simulink model "programming_simulink_bench"  (R2021b)
settings: Solver=ode1  StartTime=0.0  StopTime=120  FixedStep=0.01  RelTol=1e-3  EnableMultiTasking=on
undefined symbols (not defined in the file): a, b, c, ki, kp
libraries: arduinolib x12, arduinosensorlib x3
settings Model: ExtModeTrigDuration=2  Creator=Admin  LastModifiedBy=ASUS
settings SolverCC: AlgebraicLoopSolver=TrustRegion
settings OptimizationCC: EnhancedBackFolding=on  PassReuseOutputArgsAs=Individual arguments  ZeroExternalMemoryAtStartup=off  ZeroInternalMemoryAtStartup=off  MaxStackSize=64  OptimizeBlockOrder=speed  DifferentSizesBufferReuse=on  OptimizationCustomize=off  EfficientTunableParamExpr=on
settings DebuggingCC: ParameterTunabilityLossMsg=error  SFMachineParentedDataDiag=warning
settings HardwareCC: ProdBitPerInt=16  ProdBitPerPointer=16  ProdBitPerSizeT=16  ProdBitPerPtrDiffT=16  ProdLargestAtomicFloat=None  ProdWordSize=8  ProdHWDeviceType=Atmel->AVR
settings SFSimCC: MATLABDynamicMemAlloc=off
settings RTWCC: Description=Embedded Coder  SystemTargetFile=ert.tlc  HardwareBoard=Arduino Mega 2560  TemplateMakefile=ert_default_tmf  Toolchain=Arduino AVR  BuildConfiguration=Faster Runs
settings CodeAppCC: ForceParamTrailComments=on  IgnoreCustomStorageClasses=off  OperatorAnnotations=on  SimulinkDataObjDesc=on  SFDataObjDesc=on  InsertBlockDesc=on
settings ERTTargetCC: SupportContinuousTime=on  SupportNonInlinedSFcns=on  SupportVariableSizeSignals=on  ExtModeTransport=3  ExtModeStaticAlloc=on  ExtModeStaticAllocSize=2048  ExtModeMexFile=ext_xcp  ExtModeIntrfLevel=Level2 - Open

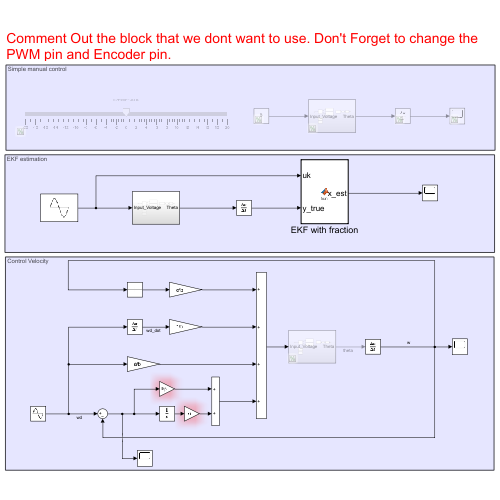
[thumbnail: Simulink's stored preview of the top-level diagram]
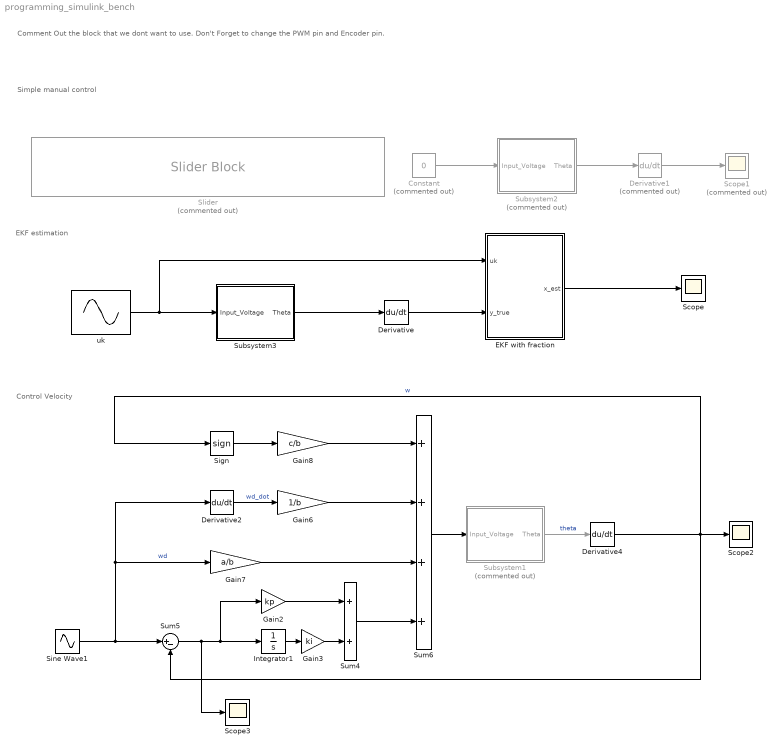
== system programming_simulink_bench ==
  note: Control Velocity
  note: Comment Out the block that we dont want to use. Don't Forget to change the PWM pin and Encoder pin.
  note: EKF estimation
  note: Simple manual control
  Constant : Constant  Commented=on  Value=0
  Derivative : Derivative
  Derivative1 : Derivative  Commented=on
  Derivative2 : Derivative
  Derivative4 : Derivative
  EKF with fraction : MATLAB Function  TreatAsAtomicUnit=on
  Gain2 : Gain  Gain=kp
  Gain3 : Gain  Gain=ki
  Gain6 : Gain  Gain=1/b
  Gain7 : Gain  Gain=a/b
  Gain8 : Gain  Gain=c/b
  Integrator1 : Integrator
  Scope : Scope
  Scope1 : Scope  Commented=on
  Scope2 : Scope
  Scope3 : Scope
  Sign : Signum
  Sine Wave1 : Sin  Amplitude=10  Frequency=2*pi*0.1  SampleTime=0
  Slider : SliderBlock  Commented=on  ScaleMin=-20  ScaleMax=20  TickInterval=2
  Subsystem1 : Subsystem  Commented=on
  Subsystem2 : Subsystem  Commented=on
  Subsystem3 : Subsystem
  Sum4 : Sum
  Sum5 : Sum  Inputs=|+-
  Sum6 : Sum  Inputs=++++
  uk : Sin  Amplitude=20  Frequency=2*pi*0.4  SampleTime=0
  wires:
  EKF with fraction/1(x_est) -> Scope/1
  Derivative/1 -> EKF with fraction/2(y_true)
  Subsystem3/1(Theta) -> Derivative/1
  uk/1 -> EKF with fraction/1(uk), Subsystem3/1(Input_Voltage)
  Constant/1 -> Subsystem2/1(Input_Voltage)
  Subsystem2/1(Theta) -> Derivative1/1
  Derivative1/1 -> Scope1/1
  Sign/1 -> Gain8/1
  Subsystem1/1(Theta) -> Derivative4/1  "theta"
  Gain6/1 -> Sum6/2
  Sum6/1 -> Subsystem1/1(Input_Voltage)
  Integrator1/1 -> Gain3/1
  Sum4/1 -> Sum6/4
  Gain8/1 -> Sum6/1
  Gain2/1 -> Sum4/1
  Sum5/1 -> Gain2/1, Integrator1/1, Scope3/1
  Derivative4/1 -> Sign/1, Sum5/2, Scope2/1  "w"
  Gain7/1 -> Sum6/3
  Sine Wave1/1 -> Sum5/1, Gain7/1, Derivative2/1  "wd"
  Gain3/1 -> Sum4/2
  Derivative2/1 -> Gain6/1  "wd_dot"

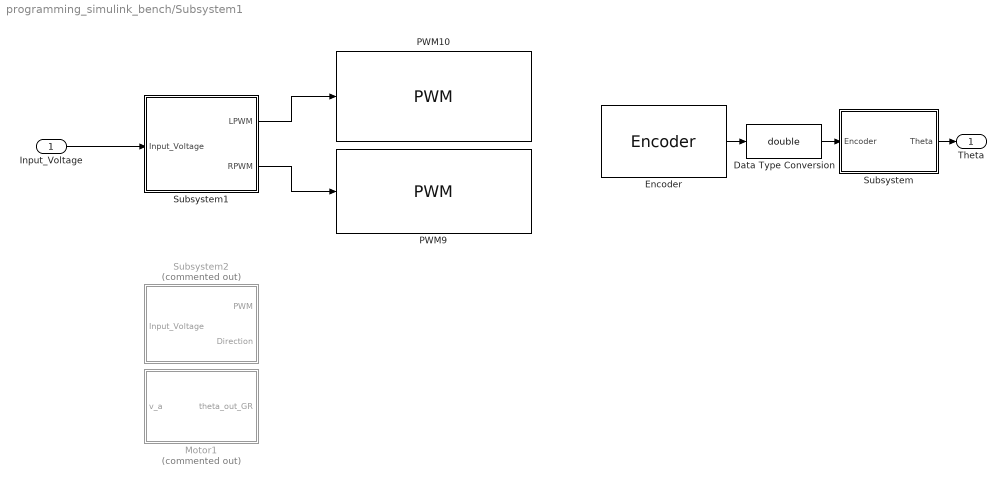
== system programming_simulink_bench/Subsystem1 ==
  Input_Voltage : Inport
  Data Type Conversion : DataTypeConversion  OutDataTypeStr=double
  Encoder : arduinosensorlib/Encoder  InputA=2  InputB=3  Mode=No reset  SampleTime=-1
      settings: SourceProductBaseCode=ARDUINO
  Motor1 : Subsystem  Commented=on
  PWM10 : arduinolib/PWM  pinNumber=8  frequencyType=Default  desiredFrequency=490.2  achievableFrequency=490.2
  PWM9 : arduinolib/PWM  pinNumber=9  frequencyType=Default  desiredFrequency=490.2  achievableFrequency=490.2
  Subsystem : Subsystem  mask(Encoder Pulse to Radian Conversion){PPR=11, Mode=1, GR=515}
      mask prompts: PPR "Base Pulse per Revolution :"; Mode "Encoder Count Mode :"; GR "Gear Box Ratio :"
      mask help: This block is used for converting motor encoder pulse to shaft position theta.
      mask TypeOptions Mode: 1 | 2 | 4
  Subsystem1 : Subsystem  mask(Motor PWM Calculation for Left, Right PWM Type){max_pwm_pulse=254, voltage_max=23.5}
      mask prompts: max_pwm_pulse "Max PWM Pulse Number :"; voltage_max "Max Voltage :"
      mask help:
      | This block is used the calculate the PWM from the input voltage for motor driver with Left and Right PWM Type (IBT-2).
      |
      | - Max PWM Pulse Number used for selecting the maximum pulse for PWM. Some driver has 255 as the maximum PWM and some has 254 as the maximum.
      |
      | - Max Voltage used for input the maximum voltage for the battery and the motor. Typically, the DC Motor and battery use 24v.
      mask TypeOptions max_pwm_pulse: 254 | 255
  Subsystem2 : Subsystem  Commented=on  mask(Motor PWM Calculation for PWM, Direction Type){max_pwm_pulse=254, voltage_max=0}
      mask help:
      | This block is used the calculate the PWM from the input voltage for motor driver with PWM and Direction Type.
      |
      | - Max PWM Pulse Number used for selecting the maximum pulse for PWM. Some driver has 255 as the maximum PWM and some has 254 as the maximum.
      |
      | - Max Voltage used for input the maximum voltage for the battery and the motor. Typically, the DC Motor and battery use 24v.
      mask TypeOptions max_pwm_pulse: 254 | 255
  Theta : Outport
  wires:
  Subsystem/1(Theta) -> Theta/1
  Subsystem1/2(RPWM) -> PWM9/1
  Input_Voltage/1 -> Subsystem1/1(Input_Voltage)
  Subsystem1/1(LPWM) -> PWM10/1
  Encoder/1 -> Data Type Conversion/1
  Data Type Conversion/1 -> Subsystem/1(Encoder)

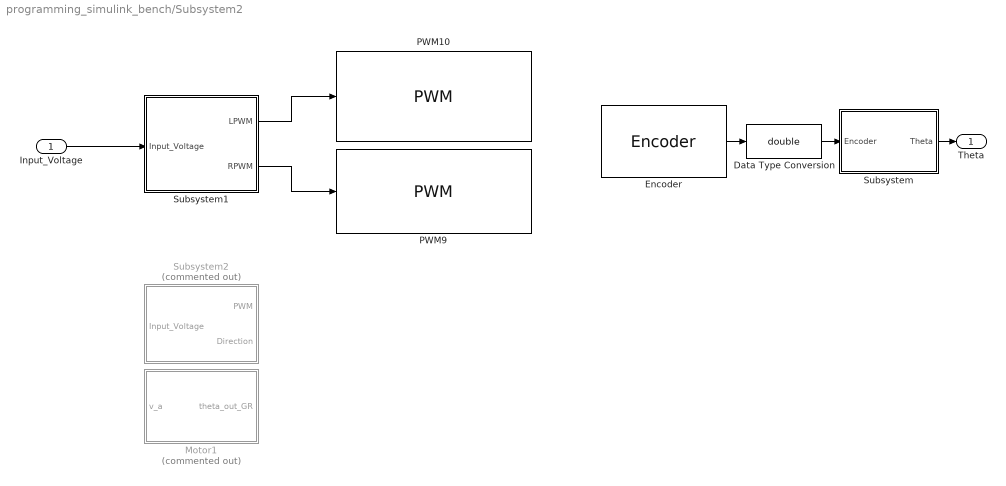
== system programming_simulink_bench/Subsystem2 ==
  Input_Voltage : Inport
  Data Type Conversion : DataTypeConversion  OutDataTypeStr=double
  Encoder : arduinosensorlib/Encoder  InputA=2  InputB=3  Mode=No reset  SampleTime=-1
      settings: SourceProductBaseCode=ARDUINO
  Motor1 : Subsystem  Commented=on
  PWM10 : arduinolib/PWM  pinNumber=8  frequencyType=Default  desiredFrequency=490.2  achievableFrequency=490.2
  PWM9 : arduinolib/PWM  pinNumber=9  frequencyType=Default  desiredFrequency=490.2  achievableFrequency=490.2
  Subsystem : Subsystem  mask(Encoder Pulse to Radian Conversion){PPR=11, Mode=1, GR=515}
      mask prompts: PPR "Base Pulse per Revolution :"; Mode "Encoder Count Mode :"; GR "Gear Box Ratio :"
      mask help: This block is used for converting motor encoder pulse to shaft position theta.
      mask TypeOptions Mode: 1 | 2 | 4
  Subsystem1 : Subsystem  mask(Motor PWM Calculation for Left, Right PWM Type){max_pwm_pulse=254, voltage_max=23.5}
      mask prompts: max_pwm_pulse "Max PWM Pulse Number :"; voltage_max "Max Voltage :"
      mask help:
      | This block is used the calculate the PWM from the input voltage for motor driver with Left and Right PWM Type (IBT-2).
      |
      | - Max PWM Pulse Number used for selecting the maximum pulse for PWM. Some driver has 255 as the maximum PWM and some has 254 as the maximum.
      |
      | - Max Voltage used for input the maximum voltage for the battery and the motor. Typically, the DC Motor and battery use 24v.
      mask TypeOptions max_pwm_pulse: 254 | 255
  Subsystem2 : Subsystem  Commented=on  mask(Motor PWM Calculation for PWM, Direction Type){max_pwm_pulse=254, voltage_max=0}
      mask help:
      | This block is used the calculate the PWM from the input voltage for motor driver with PWM and Direction Type.
      |
      | - Max PWM Pulse Number used for selecting the maximum pulse for PWM. Some driver has 255 as the maximum PWM and some has 254 as the maximum.
      |
      | - Max Voltage used for input the maximum voltage for the battery and the motor. Typically, the DC Motor and battery use 24v.
      mask TypeOptions max_pwm_pulse: 254 | 255
  Theta : Outport
  wires:
  Data Type Conversion/1 -> Subsystem/1(Encoder)
  Encoder/1 -> Data Type Conversion/1
  Subsystem1/1(LPWM) -> PWM10/1
  Input_Voltage/1 -> Subsystem1/1(Input_Voltage)
  Subsystem1/2(RPWM) -> PWM9/1
  Subsystem/1(Theta) -> Theta/1

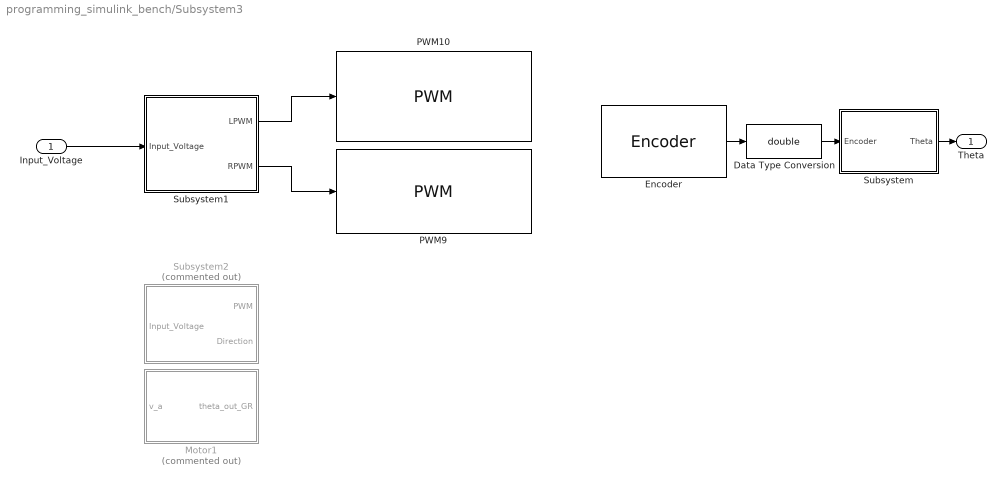
== system programming_simulink_bench/Subsystem3 ==
  Input_Voltage : Inport
  Data Type Conversion : DataTypeConversion  OutDataTypeStr=double
  Encoder : arduinosensorlib/Encoder  InputA=2  InputB=3  Mode=No reset  SampleTime=-1
      settings: SourceProductBaseCode=ARDUINO
  Motor1 : Subsystem  Commented=on
  PWM10 : arduinolib/PWM  pinNumber=8  frequencyType=Default  desiredFrequency=490.2  achievableFrequency=490.2
  PWM9 : arduinolib/PWM  pinNumber=9  frequencyType=Default  desiredFrequency=490.2  achievableFrequency=490.2
  Subsystem : Subsystem  mask(Encoder Pulse to Radian Conversion){PPR=11, Mode=1, GR=515}
      mask prompts: PPR "Base Pulse per Revolution :"; Mode "Encoder Count Mode :"; GR "Gear Box Ratio :"
      mask help: This block is used for converting motor encoder pulse to shaft position theta.
      mask TypeOptions Mode: 1 | 2 | 4
  Subsystem1 : Subsystem  mask(Motor PWM Calculation for Left, Right PWM Type){max_pwm_pulse=254, voltage_max=23.5}
      mask prompts: max_pwm_pulse "Max PWM Pulse Number :"; voltage_max "Max Voltage :"
      mask help:
      | This block is used the calculate the PWM from the input voltage for motor driver with Left and Right PWM Type (IBT-2).
      |
      | - Max PWM Pulse Number used for selecting the maximum pulse for PWM. Some driver has 255 as the maximum PWM and some has 254 as the maximum.
      |
      | - Max Voltage used for input the maximum voltage for the battery and the motor. Typically, the DC Motor and battery use 24v.
      mask TypeOptions max_pwm_pulse: 254 | 255
  Subsystem2 : Subsystem  Commented=on  mask(Motor PWM Calculation for PWM, Direction Type){max_pwm_pulse=254, voltage_max=0}
      mask help:
      | This block is used the calculate the PWM from the input voltage for motor driver with PWM and Direction Type.
      |
      | - Max PWM Pulse Number used for selecting the maximum pulse for PWM. Some driver has 255 as the maximum PWM and some has 254 as the maximum.
      |
      | - Max Voltage used for input the maximum voltage for the battery and the motor. Typically, the DC Motor and battery use 24v.
      mask TypeOptions max_pwm_pulse: 254 | 255
  Theta : Outport
  wires:
  Data Type Conversion/1 -> Subsystem/1(Encoder)
  Encoder/1 -> Data Type Conversion/1
  Subsystem1/1(LPWM) -> PWM10/1
  Input_Voltage/1 -> Subsystem1/1(Input_Voltage)
  Subsystem1/2(RPWM) -> PWM9/1
  Subsystem/1(Theta) -> Theta/1

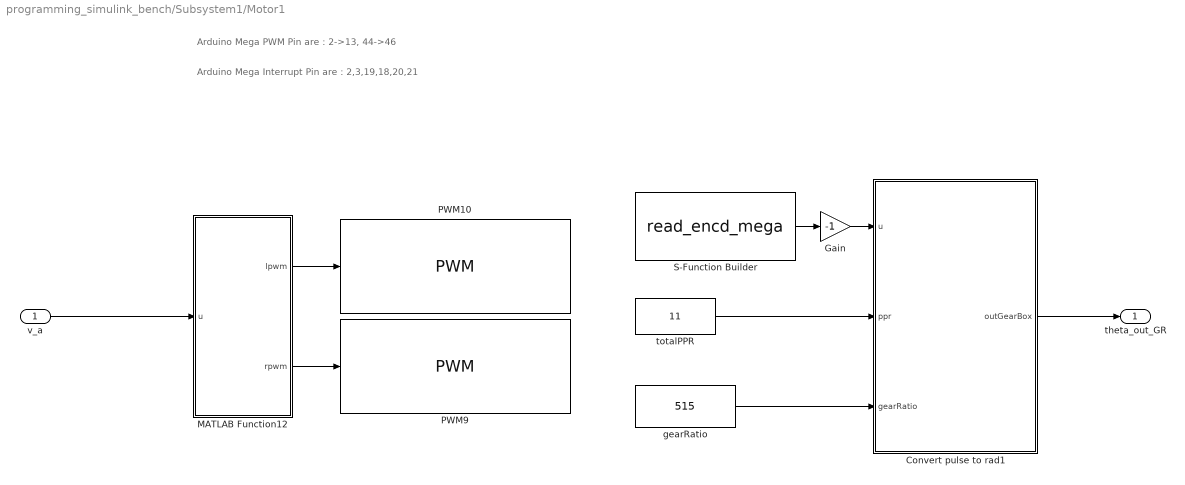
== system programming_simulink_bench/Subsystem1/Motor1 ==
  note: Arduino Mega PWM Pin are : 2->13, 44->46
  note: Arduino Mega Interrupt Pin are : 2,3,19,18,20,21
  v_a : Inport
  Convert pulse to rad1 : MATLAB Function  TreatAsAtomicUnit=on
  Gain : Gain  Gain=-1
  MATLAB Function12 : MATLAB Function  TreatAsAtomicUnit=on
  PWM10 : arduinolib/PWM  pinNumber=8  frequencyType=Default  desiredFrequency=490.2  achievableFrequency=490.2
  PWM9 : arduinolib/PWM  pinNumber=9  frequencyType=Default  desiredFrequency=490.2  achievableFrequency=490.2
  S-Function Builder : S-Function  FunctionName=read_encd_mega  SFunctionModules=read_encd_mega_wrapper  SFunctionDeploymentMode=off  EnableBusSupport=off  mask(S-Function Builder){}
      mask help: Simulink:masks:SFunctionBuilder_MD
      mask init:
      | val = [[.9  0.75 0.75 1 1 .9 .9 1]',[1 1 0.75 0.75 .9 .9 1 .9]'];try , sys = get_param(gcb,'SfunBuilderFcnName');if isempty(sys), sys = get_param(gcb,'FunctionName'); end,catch, sys = get_param(gcb,'FunctionName'); end
      settings: CopyFcn=set_param(gcbh,'LinkStatus','none')  OpenFcn=sfunctionwizard(gcbh)
      mask Display: plot(val(:,1),val(:,2)),disp(sys),port_label('output',1,'count')
  gearRatio : Constant  Value=515
  totalPPR : Constant  Value=11
  theta_out_GR : Outport
  wires:
  Gain/1 -> Convert pulse to rad1/1(u)
  S-Function Builder/1 -> Gain/1
  Convert pulse to rad1/1(outGearBox) -> theta_out_GR/1
  v_a/1 -> MATLAB Function12/1(u)
  gearRatio/1 -> Convert pulse to rad1/3(gearRatio)
  MATLAB Function12/2(rpwm) -> PWM9/1
  totalPPR/1 -> Convert pulse to rad1/2(ppr)
  MATLAB Function12/1(lpwm) -> PWM10/1

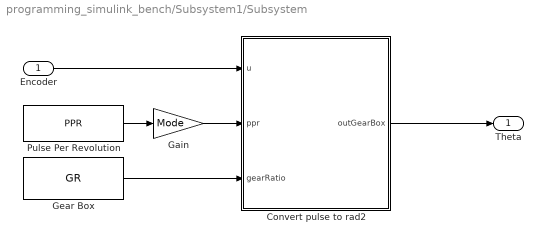
== system programming_simulink_bench/Subsystem1/Subsystem ==
  Encoder : Inport
  Convert pulse to rad2 : MATLAB Function  TreatAsAtomicUnit=on
  Gain : Gain  Gain=Mode
  Gear Box : Constant  Value=GR
  Pulse Per Revolution : Constant  Value=PPR
  Theta : Outport
  wires:
  Gain/1 -> Convert pulse to rad2/2(ppr)
  Encoder/1 -> Convert pulse to rad2/1(u)
  Gear Box/1 -> Convert pulse to rad2/3(gearRatio)
  Pulse Per Revolution/1 -> Gain/1
  Convert pulse to rad2/1(outGearBox) -> Theta/1

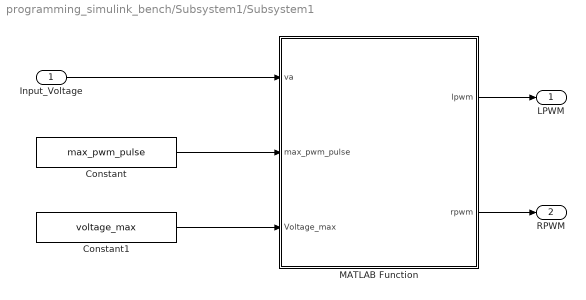
== system programming_simulink_bench/Subsystem1/Subsystem1 ==
  Input_Voltage : Inport
  Constant : Constant  Value=max_pwm_pulse
  Constant1 : Constant  Value=voltage_max
  MATLAB Function : MATLAB Function  TreatAsAtomicUnit=on
  LPWM : Outport
  RPWM : Outport  Port=2
  wires:
  Input_Voltage/1 -> MATLAB Function/1(va)
  MATLAB Function/1(lpwm) -> LPWM/1
  Constant1/1 -> MATLAB Function/3(Voltage_max)
  Constant/1 -> MATLAB Function/2(max_pwm_pulse)
  MATLAB Function/2(rpwm) -> RPWM/1

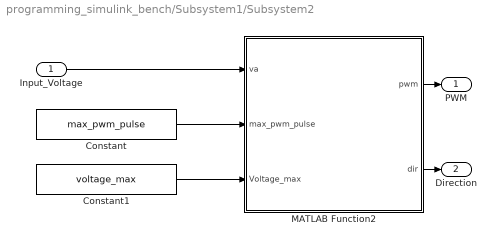
== system programming_simulink_bench/Subsystem1/Subsystem2 ==
  Input_Voltage : Inport
  Constant : Constant  Value=max_pwm_pulse
  Constant1 : Constant  Value=voltage_max
  MATLAB Function2 : MATLAB Function  TreatAsAtomicUnit=on
  PWM : Outport
  Direction : Outport  Port=2
  wires:
  MATLAB Function2/1(pwm) -> PWM/1
  Input_Voltage/1 -> MATLAB Function2/1(va)
  MATLAB Function2/2(dir) -> Direction/1
  Constant1/1 -> MATLAB Function2/3(Voltage_max)
  Constant/1 -> MATLAB Function2/2(max_pwm_pulse)

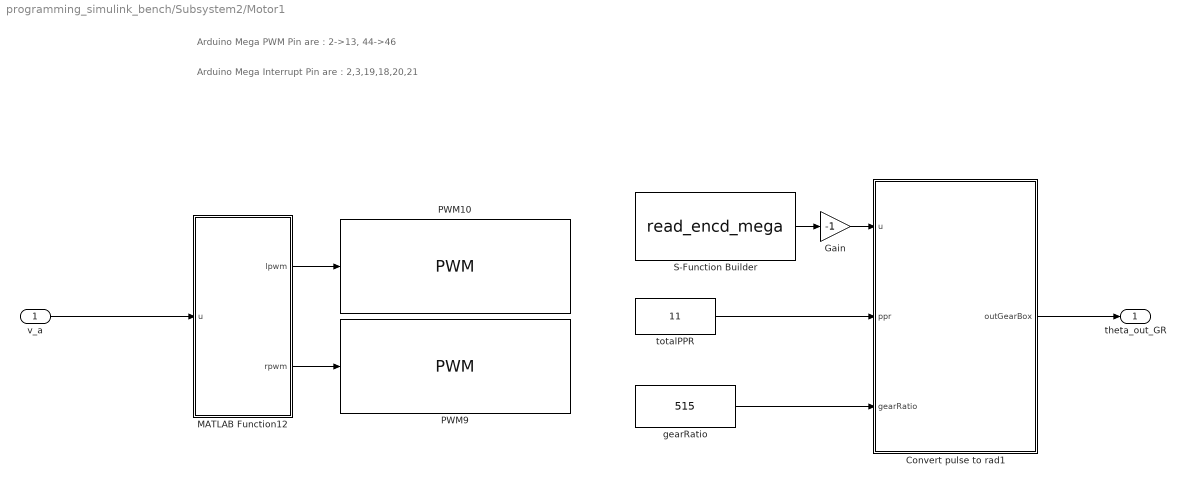
== system programming_simulink_bench/Subsystem2/Motor1 ==
  note: Arduino Mega Interrupt Pin are : 2,3,19,18,20,21
  note: Arduino Mega PWM Pin are : 2->13, 44->46
  v_a : Inport
  Convert pulse to rad1 : MATLAB Function  TreatAsAtomicUnit=on
  Gain : Gain  Gain=-1
  MATLAB Function12 : MATLAB Function  TreatAsAtomicUnit=on
  PWM10 : arduinolib/PWM  pinNumber=8  frequencyType=Default  desiredFrequency=490.2  achievableFrequency=490.2
  PWM9 : arduinolib/PWM  pinNumber=9  frequencyType=Default  desiredFrequency=490.2  achievableFrequency=490.2
  S-Function Builder : S-Function  FunctionName=read_encd_mega  SFunctionModules=read_encd_mega_wrapper  SFunctionDeploymentMode=off  EnableBusSupport=off  mask(S-Function Builder){}
      mask help: Simulink:masks:SFunctionBuilder_MD
      mask init: same as programming_simulink_bench/Subsystem1/Motor1/S-Function Builder
      settings: CopyFcn=set_param(gcbh,'LinkStatus','none')  OpenFcn=sfunctionwizard(gcbh)
      mask Display: plot(val(:,1),val(:,2)),disp(sys),port_label('output',1,'count')
  gearRatio : Constant  Value=515
  totalPPR : Constant  Value=11
  theta_out_GR : Outport
  wires:
  MATLAB Function12/1(lpwm) -> PWM10/1
  totalPPR/1 -> Convert pulse to rad1/2(ppr)
  MATLAB Function12/2(rpwm) -> PWM9/1
  gearRatio/1 -> Convert pulse to rad1/3(gearRatio)
  v_a/1 -> MATLAB Function12/1(u)
  Convert pulse to rad1/1(outGearBox) -> theta_out_GR/1
  S-Function Builder/1 -> Gain/1
  Gain/1 -> Convert pulse to rad1/1(u)

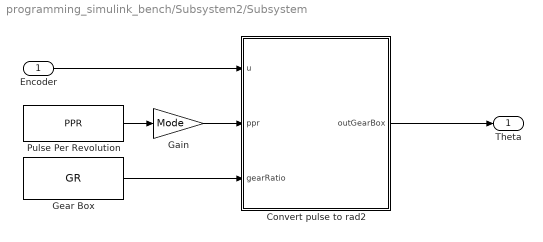
== system programming_simulink_bench/Subsystem2/Subsystem ==
  Encoder : Inport
  Convert pulse to rad2 : MATLAB Function  TreatAsAtomicUnit=on
  Gain : Gain  Gain=Mode
  Gear Box : Constant  Value=GR
  Pulse Per Revolution : Constant  Value=PPR
  Theta : Outport
  wires:
  Convert pulse to rad2/1(outGearBox) -> Theta/1
  Pulse Per Revolution/1 -> Gain/1
  Gear Box/1 -> Convert pulse to rad2/3(gearRatio)
  Encoder/1 -> Convert pulse to rad2/1(u)
  Gain/1 -> Convert pulse to rad2/2(ppr)

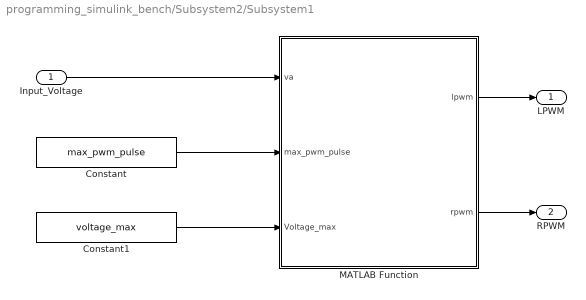
== system programming_simulink_bench/Subsystem2/Subsystem1 ==
  Input_Voltage : Inport
  Constant : Constant  Value=max_pwm_pulse
  Constant1 : Constant  Value=voltage_max
  MATLAB Function : MATLAB Function  TreatAsAtomicUnit=on
  LPWM : Outport
  RPWM : Outport  Port=2
  wires:
  MATLAB Function/2(rpwm) -> RPWM/1
  Constant/1 -> MATLAB Function/2(max_pwm_pulse)
  Constant1/1 -> MATLAB Function/3(Voltage_max)
  MATLAB Function/1(lpwm) -> LPWM/1
  Input_Voltage/1 -> MATLAB Function/1(va)

== system programming_simulink_bench/Subsystem2/Subsystem2 ==
  Input_Voltage : Inport
  Constant : Constant  Value=max_pwm_pulse
  Constant1 : Constant  Value=voltage_max
  MATLAB Function2 : MATLAB Function  TreatAsAtomicUnit=on
  PWM : Outport
  Direction : Outport  Port=2
  wires:
  Constant/1 -> MATLAB Function2/2(max_pwm_pulse)
  Constant1/1 -> MATLAB Function2/3(Voltage_max)
  MATLAB Function2/2(dir) -> Direction/1
  Input_Voltage/1 -> MATLAB Function2/1(va)
  MATLAB Function2/1(pwm) -> PWM/1

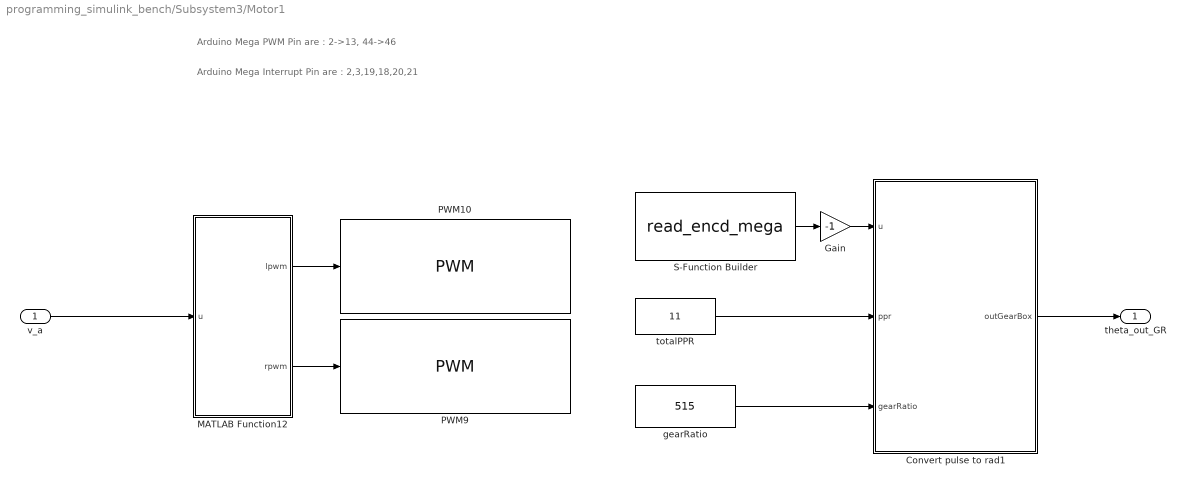
== system programming_simulink_bench/Subsystem3/Motor1 ==
  note: Arduino Mega Interrupt Pin are : 2,3,19,18,20,21
  note: Arduino Mega PWM Pin are : 2->13, 44->46
  v_a : Inport
  Convert pulse to rad1 : MATLAB Function  TreatAsAtomicUnit=on
  Gain : Gain  Gain=-1
  MATLAB Function12 : MATLAB Function  TreatAsAtomicUnit=on
  PWM10 : arduinolib/PWM  pinNumber=8  frequencyType=Default  desiredFrequency=490.2  achievableFrequency=490.2
  PWM9 : arduinolib/PWM  pinNumber=9  frequencyType=Default  desiredFrequency=490.2  achievableFrequency=490.2
  S-Function Builder : S-Function  FunctionName=read_encd_mega  SFunctionModules=read_encd_mega_wrapper  SFunctionDeploymentMode=off  EnableBusSupport=off  mask(S-Function Builder){}
      mask help: Simulink:masks:SFunctionBuilder_MD
      mask init: same as programming_simulink_bench/Subsystem1/Motor1/S-Function Builder
      settings: CopyFcn=set_param(gcbh,'LinkStatus','none')  OpenFcn=sfunctionwizard(gcbh)
      mask Display: plot(val(:,1),val(:,2)),disp(sys),port_label('output',1,'count')
  gearRatio : Constant  Value=515
  totalPPR : Constant  Value=11
  theta_out_GR : Outport
  wires:
  MATLAB Function12/1(lpwm) -> PWM10/1
  totalPPR/1 -> Convert pulse to rad1/2(ppr)
  MATLAB Function12/2(rpwm) -> PWM9/1
  gearRatio/1 -> Convert pulse to rad1/3(gearRatio)
  v_a/1 -> MATLAB Function12/1(u)
  Convert pulse to rad1/1(outGearBox) -> theta_out_GR/1
  S-Function Builder/1 -> Gain/1
  Gain/1 -> Convert pulse to rad1/1(u)

== system programming_simulink_bench/Subsystem3/Subsystem ==
  Encoder : Inport
  Convert pulse to rad2 : MATLAB Function  TreatAsAtomicUnit=on
  Gain : Gain  Gain=Mode
  Gear Box : Constant  Value=GR
  Pulse Per Revolution : Constant  Value=PPR
  Theta : Outport
  wires:
  Convert pulse to rad2/1(outGearBox) -> Theta/1
  Pulse Per Revolution/1 -> Gain/1
  Gear Box/1 -> Convert pulse to rad2/3(gearRatio)
  Encoder/1 -> Convert pulse to rad2/1(u)
  Gain/1 -> Convert pulse to rad2/2(ppr)

== system programming_simulink_bench/Subsystem3/Subsystem1 ==
  Input_Voltage : Inport
  Constant : Constant  Value=max_pwm_pulse
  Constant1 : Constant  Value=voltage_max
  MATLAB Function : MATLAB Function  TreatAsAtomicUnit=on
  LPWM : Outport
  RPWM : Outport  Port=2
  wires:
  MATLAB Function/2(rpwm) -> RPWM/1
  Constant/1 -> MATLAB Function/2(max_pwm_pulse)
  Constant1/1 -> MATLAB Function/3(Voltage_max)
  MATLAB Function/1(lpwm) -> LPWM/1
  Input_Voltage/1 -> MATLAB Function/1(va)

== system programming_simulink_bench/Subsystem3/Subsystem2 ==
  Input_Voltage : Inport
  Constant : Constant  Value=max_pwm_pulse
  Constant1 : Constant  Value=voltage_max
  MATLAB Function2 : MATLAB Function  TreatAsAtomicUnit=on
  PWM : Outport
  Direction : Outport  Port=2
  wires:
  Constant/1 -> MATLAB Function2/2(max_pwm_pulse)
  Constant1/1 -> MATLAB Function2/3(Voltage_max)
  MATLAB Function2/2(dir) -> Direction/1
  Input_Voltage/1 -> MATLAB Function2/1(va)
  MATLAB Function2/1(pwm) -> PWM/1

== matlab function programming_simulink_bench/Subsystem1/Subsystem2/MATLAB Function2 ==
  data: va input; pwm output; dir output; max_pwm_pulse input; Voltage_max input
function [pwm,dir] = fcn(va,max_pwm_pulse,Voltage_max)

pwm_cal = va*max_pwm_pulse/Voltage_max;
if pwm_cal > 0
    pwm = pwm_cal;
    dir = 0;
elseif pwm_cal < 0
    pwm = abs(pwm_cal);
    dir = 1;
else
    pwm = 0;
    dir = 0;
end

== matlab function programming_simulink_bench/Subsystem2/Motor1/Convert pulse to rad1 ==
  settings: updateMethod=DISCRETE
  data: u input; ppr input; gearRatio input; outGearBox output
function outGearBox = fcn(u,ppr,gearRatio)

persistent counter_num over_flag
if(isempty(counter_num)), counter_num = 0;end
if(isempty(over_flag)), over_flag = 0;end
pulse2radian = 2*pi/ppr; % 1 pulse = ?? radian

if(double(u) - counter_num > 40000), over_flag = over_flag-1;
elseif(double(u) - counter_num < -40000), over_flag = over_flag+1;
end

inGearBox = (double(u)+over_flag*(2^32 -1))*pulse2radian; 
outGearBox = inGearBox/gearRatio;
counter_num = double(u) ;

== matlab function programming_simulink_bench/EKF with fraction ==
  settings: updateMethod=DISCRETE
  data: uk input; y_true input; x_est output
function x_est = fcn(uk,y_true)
Ts=0.01;
persistent x_est_p P Qd_est R_est Qc_est;
if isempty(x_est_p)
          
          x_est_p=[2;13;25;1];
          P=2*eye(4);
         Qc_est=1e-5*diag([10,25,25,1]);
          Qd_est=Qc_est*Ts;
          R_est=0.02;
end
c=[1 0 0 0];D=0;Ck=c;Dk=D;
%Comput Kalman Gain and update predicted value
Wk=P*Ck'/(Ck*P*Ck'+R_est);
y_est=Ck*x_est_p+Dk*uk;
x=x_est_p+Wk.*(y_true-y_est);
%Compute prediction at next time step
x_est=x+Ts*[-x(2)*x(1)+uk*x(3)-x(4)*sign(x(1));0;0;0];
%Update error covariance matrices
P=P-Wk*Ck*P;
%Define Ak
Ak=eye(4)+Ts*[-x(2) -x(1) uk -sign(x(1));0 0 0 0;0 0 0 0;0 0 0 0];
P=Ak*P*Ak'+Qd_est;
x_est_p=x_est;

== matlab function programming_simulink_bench/Subsystem2/Motor1/MATLAB Function12 ==
  data: u input; lpwm output; rpwm output
function [lpwm,rpwm] = fcn(u)

Vmax = 23.5;
pwm = u*254/Vmax;
if pwm > 0
    lpwm = pwm;
    rpwm = 0;
elseif pwm < 0
    lpwm = 0;
    rpwm = abs(pwm);
else
    lpwm = 0;
    rpwm = 0;
end

== matlab function programming_simulink_bench/Subsystem2/Subsystem/Convert pulse to rad2 ==
  settings: updateMethod=DISCRETE
  data: u input; ppr input; gearRatio input; outGearBox output
function outGearBox = fcn(u,ppr,gearRatio)

persistent counter_num over_flag
if(isempty(counter_num)), counter_num = 0;end
if(isempty(over_flag)), over_flag = 0;end
pulse2radian = 2*pi/ppr; % 1 pulse = ?? radian

if(double(u) - counter_num > 40000), over_flag = over_flag-1;
elseif(double(u) - counter_num < -40000), over_flag = over_flag+1;
end

inGearBox = (double(u)+over_flag*(2^32 -1))*pulse2radian; 
outGearBox = inGearBox/gearRatio;
counter_num = double(u) ;

== matlab function programming_simulink_bench/Subsystem2/Subsystem1/MATLAB Function ==
  data: va input; lpwm output; max_pwm_pulse input; Voltage_max input; rpwm output
function [lpwm,rpwm] = fcn(va,max_pwm_pulse,Voltage_max)

pwm = va*max_pwm_pulse/Voltage_max;
if pwm > 0
    lpwm = pwm;
    rpwm = 0;
elseif pwm < 0
    lpwm = 0;
    rpwm = abs(pwm);
else
    lpwm = 0;
    rpwm = 0;
end

== matlab function programming_simulink_bench/Subsystem2/Subsystem2/MATLAB Function2 ==
  data: va input; pwm output; dir output; max_pwm_pulse input; Voltage_max input
function [pwm,dir] = fcn(va,max_pwm_pulse,Voltage_max)

pwm_cal = va*max_pwm_pulse/Voltage_max;
if pwm_cal > 0
    pwm = pwm_cal;
    dir = 0;
elseif pwm_cal < 0
    pwm = abs(pwm_cal);
    dir = 1;
else
    pwm = 0;
    dir = 0;
end

== matlab function programming_simulink_bench/Subsystem1/Motor1/Convert pulse to rad1 ==
  settings: updateMethod=DISCRETE
  data: u input; ppr input; gearRatio input; outGearBox output
function outGearBox = fcn(u,ppr,gearRatio)

persistent counter_num over_flag
if(isempty(counter_num)), counter_num = 0;end
if(isempty(over_flag)), over_flag = 0;end
pulse2radian = 2*pi/ppr; % 1 pulse = ?? radian

if(double(u) - counter_num > 40000), over_flag = over_flag-1;
elseif(double(u) - counter_num < -40000), over_flag = over_flag+1;
end

inGearBox = (double(u)+over_flag*(2^32 -1))*pulse2radian; 
outGearBox = inGearBox/gearRatio;
counter_num = double(u) ;

== matlab function programming_simulink_bench/Subsystem3/Motor1/Convert pulse to rad1 ==
  settings: updateMethod=DISCRETE
  data: u input; ppr input; gearRatio input; outGearBox output
function outGearBox = fcn(u,ppr,gearRatio)

persistent counter_num over_flag
if(isempty(counter_num)), counter_num = 0;end
if(isempty(over_flag)), over_flag = 0;end
pulse2radian = 2*pi/ppr; % 1 pulse = ?? radian

if(double(u) - counter_num > 40000), over_flag = over_flag-1;
elseif(double(u) - counter_num < -40000), over_flag = over_flag+1;
end

inGearBox = (double(u)+over_flag*(2^32 -1))*pulse2radian; 
outGearBox = inGearBox/gearRatio;
counter_num = double(u) ;

== matlab function programming_simulink_bench/Subsystem1/Motor1/MATLAB Function12 ==
  data: u input; lpwm output; rpwm output
function [lpwm,rpwm] = fcn(u)

Vmax = 23.5;
pwm = u*254/Vmax;
if pwm > 0
    lpwm = pwm;
    rpwm = 0;
elseif pwm < 0
    lpwm = 0;
    rpwm = abs(pwm);
else
    lpwm = 0;
    rpwm = 0;
end

== matlab function programming_simulink_bench/Subsystem3/Motor1/MATLAB Function12 ==
  data: u input; lpwm output; rpwm output
function [lpwm,rpwm] = fcn(u)

Vmax = 23.5;
pwm = u*254/Vmax;
if pwm > 0
    lpwm = pwm;
    rpwm = 0;
elseif pwm < 0
    lpwm = 0;
    rpwm = abs(pwm);
else
    lpwm = 0;
    rpwm = 0;
end

== matlab function programming_simulink_bench/Subsystem3/Subsystem/Convert pulse to rad2 ==
  settings: updateMethod=DISCRETE
  data: u input; ppr input; gearRatio input; outGearBox output
function outGearBox = fcn(u,ppr,gearRatio)

persistent counter_num over_flag
if(isempty(counter_num)), counter_num = 0;end
if(isempty(over_flag)), over_flag = 0;end
pulse2radian = 2*pi/ppr; % 1 pulse = ?? radian

if(double(u) - counter_num > 40000), over_flag = over_flag-1;
elseif(double(u) - counter_num < -40000), over_flag = over_flag+1;
end

inGearBox = (double(u)+over_flag*(2^32 -1))*pulse2radian; 
outGearBox = inGearBox/gearRatio;
counter_num = double(u) ;

== matlab function programming_simulink_bench/Subsystem3/Subsystem1/MATLAB Function ==
  data: va input; lpwm output; max_pwm_pulse input; Voltage_max input; rpwm output
function [lpwm,rpwm] = fcn(va,max_pwm_pulse,Voltage_max)

pwm = va*max_pwm_pulse/Voltage_max;
if pwm > 0
    lpwm = pwm;
    rpwm = 0;
elseif pwm < 0
    lpwm = 0;
    rpwm = abs(pwm);
else
    lpwm = 0;
    rpwm = 0;
end

== matlab function programming_simulink_bench/Subsystem3/Subsystem2/MATLAB Function2 ==
  data: va input; pwm output; dir output; max_pwm_pulse input; Voltage_max input
function [pwm,dir] = fcn(va,max_pwm_pulse,Voltage_max)

pwm_cal = va*max_pwm_pulse/Voltage_max;
if pwm_cal > 0
    pwm = pwm_cal;
    dir = 0;
elseif pwm_cal < 0
    pwm = abs(pwm_cal);
    dir = 1;
else
    pwm = 0;
    dir = 0;
end

== matlab function programming_simulink_bench/Subsystem1/Subsystem/Convert pulse to rad2 ==
  settings: updateMethod=DISCRETE
  data: u input; ppr input; gearRatio input; outGearBox output
function outGearBox = fcn(u,ppr,gearRatio)

persistent counter_num over_flag
if(isempty(counter_num)), counter_num = 0;end
if(isempty(over_flag)), over_flag = 0;end
pulse2radian = 2*pi/ppr; % 1 pulse = ?? radian

if(double(u) - counter_num > 40000), over_flag = over_flag-1;
elseif(double(u) - counter_num < -40000), over_flag = over_flag+1;
end

inGearBox = (double(u)+over_flag*(2^32 -1))*pulse2radian; 
outGearBox = inGearBox/gearRatio;
counter_num = double(u) ;

== matlab function programming_simulink_bench/Subsystem1/Subsystem1/MATLAB Function ==
  data: va input; lpwm output; max_pwm_pulse input; Voltage_max input; rpwm output
function [lpwm,rpwm] = fcn(va,max_pwm_pulse,Voltage_max)

pwm = va*max_pwm_pulse/Voltage_max;
if pwm > 0
    lpwm = pwm;
    rpwm = 0;
elseif pwm < 0
    lpwm = 0;
    rpwm = abs(pwm);
else
    lpwm = 0;
    rpwm = 0;
end
